simulink model "exp_5"  (R2013b)
settings: Solver=ode3  StartTime=0.0  StopTime=10.0  FixedStep=0.02  RelTol=1e-3
libraries: simulink x1
settings Model: Creator=lenovo  LastModifiedBy=lenovo

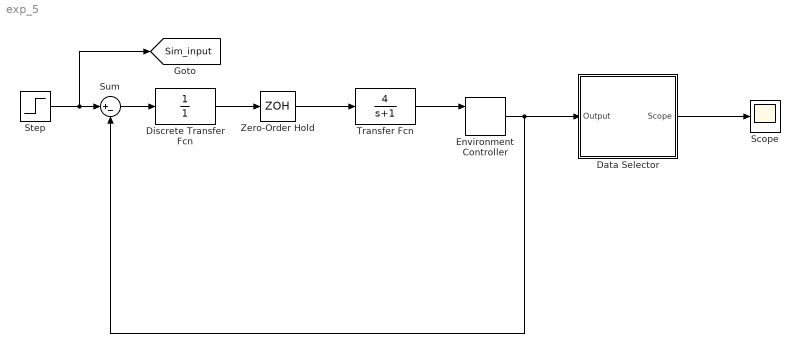
== system exp_5 ==
  "Data Selector " : Subsystem
  Discrete Transfer Fcn : DiscreteTransferFcn  Denominator=[1]  SampleTime=0.02
  Environment Controller : simulink/Signal Routing/Environment Controller
  Scope : Scope
  Step : Step  SampleTime=0
  Sum : Sum  Inputs=|+-
  Transfer Fcn : TransferFcn  Numerator=4  Denominator=[1 1]
  Zero-Order Hold : ZeroOrderHold  SampleTime=-1
  tag scope: Sim_input=global
  wires:
  Step/1 -> [Sim_input], Sum/1
  Sum/1 -> Discrete Transfer Fcn/1
  Discrete Transfer Fcn/1 -> Zero-Order Hold/1
  Zero-Order Hold/1 -> Transfer Fcn/1
  Transfer Fcn/1 -> Environment Controller/1
  Environment Controller/1 -> Sum/2, "Data Selector "/1(Output)
  "Data Selector "/1(Scope) -> Scope/1

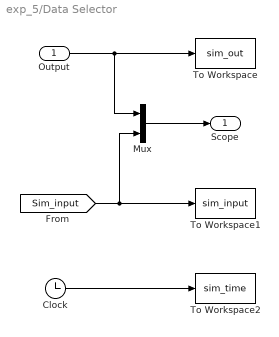
== system exp_5/Data Selector  ==
  Output : Inport
  Clock : Clock
  Mux : Mux  Inputs=2
  To Workspace : ToWorkspace  VariableName=sim_out  SampleTime=-1  SaveFormat=Timeseries
  To Workspace1 : ToWorkspace  VariableName=sim_input  SampleTime=-1  SaveFormat=Timeseries
  To Workspace2 : ToWorkspace  VariableName=sim_time  SampleTime=-1  SaveFormat=Timeseries
  Scope : Outport
  wires:
  Output/1 -> Mux/1, To Workspace/1
  Clock/1 -> To Workspace2/1
  Mux/1 -> Scope/1
  [Sim_input] -> To Workspace1/1, Mux/2
